simulink model "Project_Papi_Rubber_Game_KF_Sim"  (R2019a)
settings: Solver=FixedStepAuto  StartTime=0.0  StopTime=50  FixedStep=0.01  RelTol=1e-3
undefined symbols (not defined in the file): A, B, C, ene, init_cond, K, m, Q, R, slop
libraries: simulink x2
settings Model: Creator=asjos  LastModifiedBy=asjos

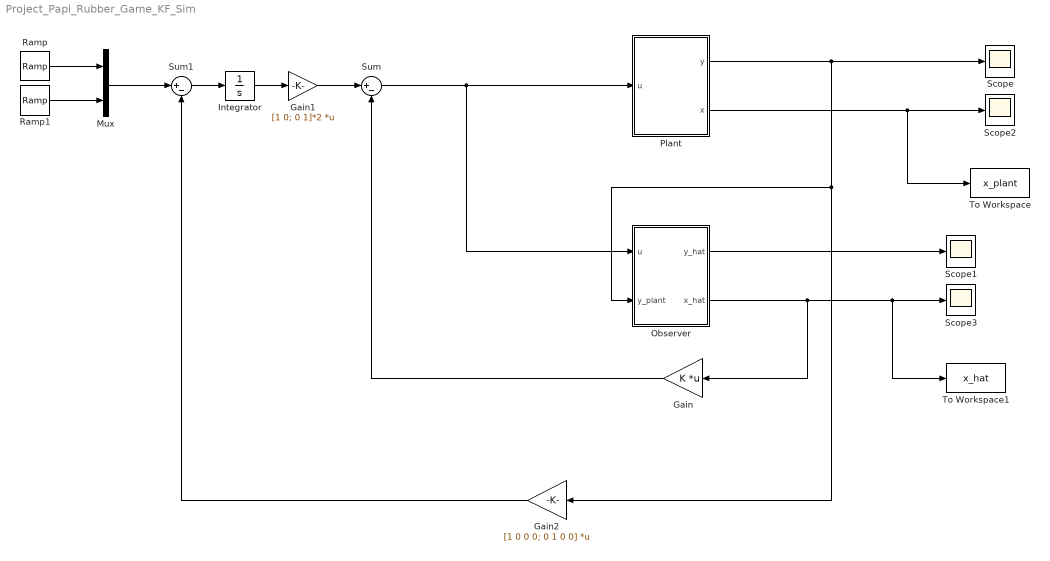
== system Project_Papi_Rubber_Game_KF_Sim ==
  Gain : Gain  Gain=K  Multiplication=Matrix(K*u)
  Gain1 : Gain  Gain=[1 0; 0 1]*2  Multiplication=Matrix(K*u)
  Gain2 : Gain  Gain=[1 0 0 0; 0 1 0 0]  Multiplication=Matrix(K*u)
  Integrator : Integrator  InitialCondition=zeros(2,1)
  Mux : Mux  Inputs=2
  Observer : Subsystem
  Plant : Subsystem
  Ramp : simulink/Sources/Ramp  slope=slop(1,m)  start=0  InitialOutput=ene(1,1)
  Ramp1 : simulink/Sources/Ramp  slope=slop(1,m)  start=0  InitialOutput=ene(1,2)
  Scope{,1..3} (4 alike) : Scope
  Sum : Sum  Inputs=|+-
  Sum1 : Sum  Inputs=|+-
  To Workspace : ToWorkspace  VariableName=x_plant  SaveFormat=Timeseries  SampleTime=-1
  To Workspace1 : ToWorkspace  VariableName=x_hat  SaveFormat=Timeseries  SampleTime=-1
  wires:
  Plant/1(y) -> Gain2/1, Observer/2(y_plant), Scope/1
  Sum/1 -> Observer/1(u), Plant/1(u)
  Gain/1 -> Sum/2
  Observer/2(x_hat) -> To Workspace1/1, Scope3/1, Gain/1
  Observer/1(y_hat) -> Scope1/1
  Plant/2(x) -> To Workspace/1, Scope2/1
  Ramp/1 -> Mux/1
  Ramp1/1 -> Mux/2
  Mux/1 -> Sum1/1
  Sum1/1 -> Integrator/1
  Gain1/1 -> Sum/1
  Integrator/1 -> Gain1/1
  Gain2/1 -> Sum1/2

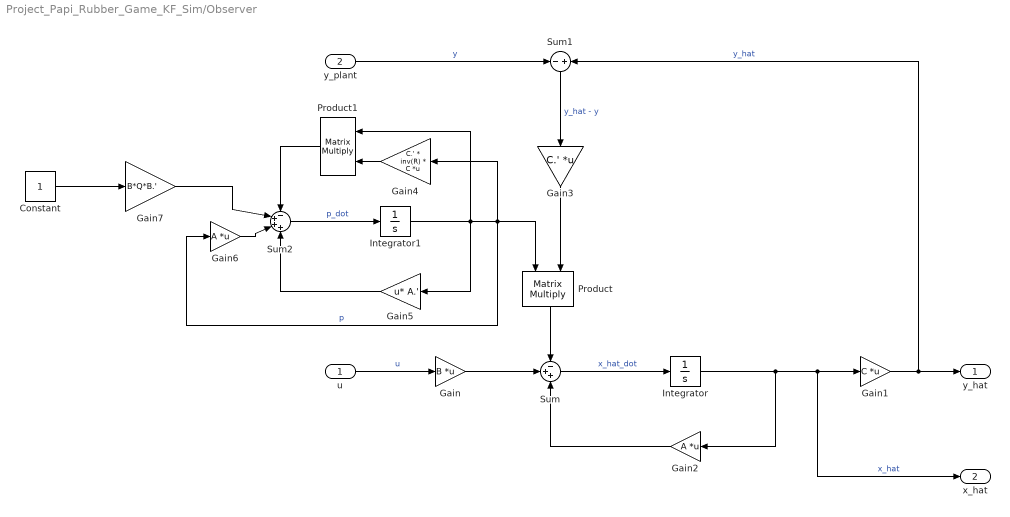
== system Project_Papi_Rubber_Game_KF_Sim/Observer ==
  u : Inport
  y_plant : Inport  Port=2
  Constant : Constant
  Gain : Gain  Gain=B  Multiplication=Matrix(K*u)
  Gain1 : Gain  Gain=C  Multiplication=Matrix(K*u)
  Gain2 : Gain  Gain=A  Multiplication=Matrix(K*u)
  Gain3 : Gain  Gain=C.'  Multiplication=Matrix(K*u)
  Gain4 : Gain  Gain=C.' * inv(R) * C  Multiplication=Matrix(K*u)
  Gain5 : Gain  Gain=A.'  Multiplication=Matrix(u*K)
  Gain6 : Gain  Gain=A  Multiplication=Matrix(K*u)
  Gain7 : Gain  Gain=B*Q*B.'
  Integrator : Integrator  InitialCondition=init_cond
  Integrator1 : Integrator  InitialCondition=50*eye(6)
  Product : Product  Multiplication=Matrix(*)
  Product1 : Product  Multiplication=Matrix(*)
  Sum : Sum  Inputs=-++
  Sum1 : Sum  Inputs=-|+
  Sum2 : Sum  Inputs=-+++
  y_hat : Outport
  x_hat : Outport  Port=2
  wires:
  Integrator/1 -> x_hat/1, Gain1/1, Gain2/1  "x_hat"
  Sum/1 -> Integrator/1  "x_hat_dot"
  u/1 -> Gain/1  "u"
  Gain1/1 -> Sum1/2, y_hat/1  "y_hat"
  Gain/1 -> Sum/2
  Gain2/1 -> Sum/3
  y_plant/1 -> Sum1/1  "y"
  Sum2/1 -> Integrator1/1  "p_dot"
  Sum1/1 -> Gain3/1  "y_hat - y"
  Gain3/1 -> Product/2
  Integrator1/1 -> Gain5/1, Product1/1, Gain4/1, Gain6/1, Product/1  "p"
  Product1/1 -> Sum2/1
  Product/1 -> Sum/1
  Gain4/1 -> Product1/2
  Gain5/1 -> Sum2/4
  Gain6/1 -> Sum2/3
  Constant/1 -> Gain7/1
  Gain7/1 -> Sum2/2

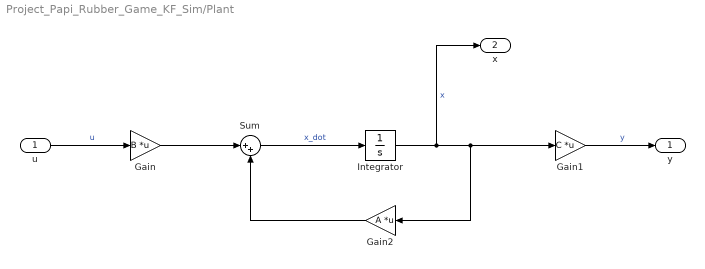
== system Project_Papi_Rubber_Game_KF_Sim/Plant ==
  u : Inport
  Gain : Gain  Gain=B  Multiplication=Matrix(K*u)
  Gain1 : Gain  Gain=C  Multiplication=Matrix(K*u)
  Gain2 : Gain  Gain=A  Multiplication=Matrix(K*u)
  Integrator : Integrator  InitialCondition=init_cond
  Sum : Sum  Inputs=|++
  y : Outport
  x : Outport  Port=2
  wires:
  Integrator/1 -> x/1, Gain1/1, Gain2/1  "x"
  Gain2/1 -> Sum/2
  Gain/1 -> Sum/1
  Sum/1 -> Integrator/1  "x_dot"
  u/1 -> Gain/1  "u"
  Gain1/1 -> y/1  "y"
